simulink model "ideal_buck_boost_non_inverter"  (R2018a)
settings: Solver=FixedStepAuto  StartTime=0.0  StopTime=1  FixedStep=Ti  RelTol=1e-3
undefined symbols (not defined in the file): A, B, Co, disturbance_Ro_enable, disturbance_Ro_time, disturbance_Vin_enable, disturbance_Vin_time, Fsw, L, opt_constant_reference, opt_pwm, opt_theorem, opt_update_equilibrium, P, pwm_limit_lower, pwm_limit_upper, pwm_pid_kd, pwm_pid_ki, pwm_pid_kp, pwm_sample_time, Q, R, Rc, reference_pid_ki, reference_pid_kp, Ro, Ro_p, sensor_sample, sys, Ti, ts, Vo, Vs, Vs_p, xe
libraries: powerlib x19, simulink x6, pePwmGenerator x1
settings Model: SimulationMode=accelerator  Creator=TARCIO-FEM  LastModifiedBy=Julio-LEPO
settings OptimizationCC: EfficientMapNaN2IntZero=off
settings HardwareCC: TargetBitPerPointer=64  TargetBitPerSizeT=64  TargetBitPerPtrDiffT=64  TargetLongLongMode=on  TargetIntDivRoundTo=Zero  TargetEndianess=LittleEndian  TargetWordSize=64  TargetHWDeviceType=MATLAB Host  ProdEqTarget=off
settings CodeAppCC: MaxIdLength=128
settings GRTTargetCC: TargetLangStandard=C89/C90 (ANSI)  CombineOutputUpdateFcns=off  GRTInterface=on

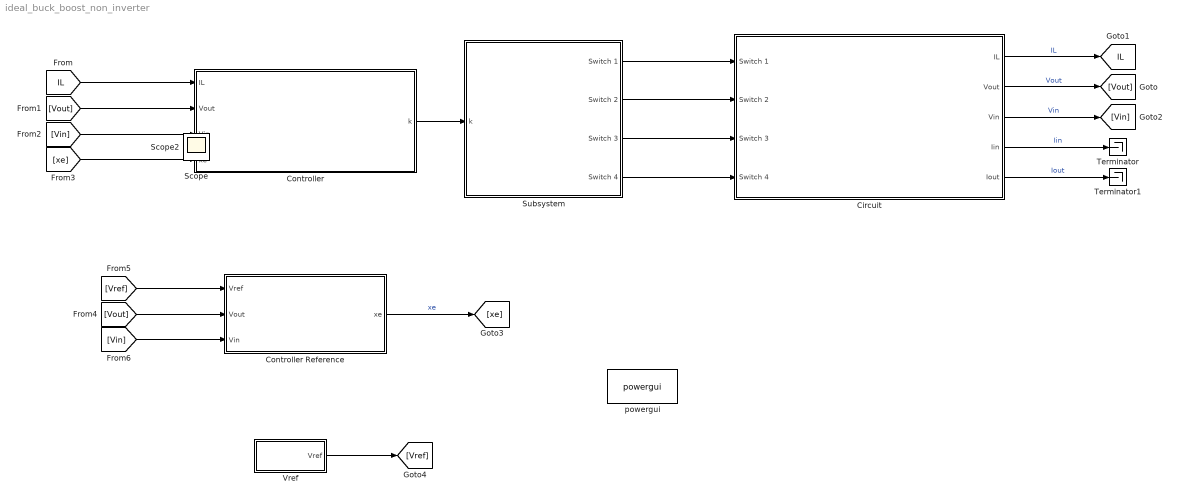
== system ideal_buck_boost_non_inverter ==
  Circuit : Subsystem
  Controller : Subsystem
  Controller Reference : Subsystem
  Subsystem : Subsystem
  Terminator : Terminator
  Terminator1 : Terminator
  Vref : Subsystem
  powergui : powerlib/powergui  Priority=1  SimulationMode=Discrete  SampleTime=Ti  frequency=60  Iterations=50  frequencyindice=0  Pbase=100e6  ErrMax=1e-4  UnitsV=kV  UnitsW=MW  buscounter=0  FunctionMessages=off  echomessages=off  EnableUseOfTLC=off  CurrentSourceSwitches=off  DisableSnubberDevices=off  DisableRonSwitches=off  DisableVfSwitches=off  DisplayEquations=off  SolverType=Tustin/Backward Euler (TBE)  Interpol=off  ExternalGateDelay=off  methode=off  Ts=100  x0status=blocks  SPID=off  SwTol=0  HookPort=off  RestoreLinks=warning  ResistiveCurrentMeasurement=off  Frange=[0:2:500]  Ylog=off  Xlog=on  ShowGrid=off  save=off  variable=ZData  structure=0  ZoomFFT=off  StartTime=0.0  cycles=1  DisplayStyle=1  fundamental=60  FreqAxis=off  MaxFrequency=1000  frequencyindicesteady=1  RmsSteady=1  display=off
  Scope : Scope
  Scope2 : Scope
  tag scope: IL=global
  wires:
  Circuit/1(IL) -> [IL]  "IL"
  Circuit/2(Vout) -> [Vout]  "Vout"
  Circuit/3(Vin) -> [Vin]  "Vin"
  [IL] -> Controller/1(IL)
  [xe] -> Controller/4(xe)
  [Vout] -> Controller Reference/2(Vout)
  [Vin] -> Controller/3(Vin)
  [Vout] -> Controller/2(Vout)
  Controller Reference/1(xe) -> [xe]  "xe"
  [Vin] -> Controller Reference/3(Vin)
  [Vref] -> Controller Reference/1(Vref)
  Vref/1(Vref) -> [Vref]
  Circuit/4(Iin) -> Terminator/1  "Iin"
  Circuit/5(Iout) -> Terminator1/1  "Iout"
  Controller/1(k) -> Subsystem/1(k)
  Subsystem/1(Switch 1) -> Circuit/1(Switch 1)
  Subsystem/2(Switch 2) -> Circuit/2(Switch 2)
  Subsystem/3(Switch 3) -> Circuit/3(Switch 3)
  Subsystem/4(Switch 4) -> Circuit/4(Switch 4)

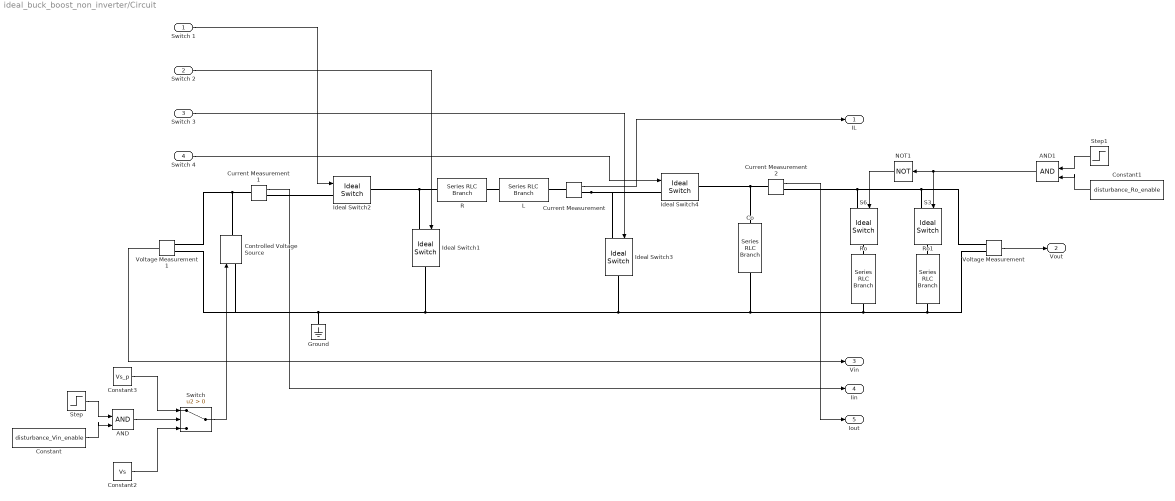
== system ideal_buck_boost_non_inverter/Circuit ==
  Switch 1 : Inport
  Switch 2 : Inport  Port=2
  Switch 3 : Inport  Port=3
  Switch 4 : Inport  Port=4
  AND : Logic  IconShape=distinctive  AllPortsSameDT=off  OutDataTypeStr=boolean
  AND1 : Logic  IconShape=distinctive  AllPortsSameDT=off  OutDataTypeStr=boolean
  Co : powerlib/Elements/Series RLC Branch  LConnTagsString=__new0  RConnTagsString=__new0  BranchType=C  Resistance=Rc  Inductance=L  SetiL0=off  InitialCurrent=0  Capacitance=Co  Setx0=off  InitialVoltage=0  Measurements=None
  Constant : Constant  Value=disturbance_Vin_enable
  Constant1 : Constant  Value=disturbance_Ro_enable
  Constant2 : Constant  Value=Vs
  Constant3 : Constant  Value=Vs_p
  Controlled Voltage Source : powerlib/Electrical Sources/Controlled Voltage Source  Initialize=on  Source_Type=DC  Amplitude=0  Phase=0  Frequency=0  Measurements=None
  Current Measurement : powerlib/Measurements/Current Measurement  PhasorSimulation=off  OutputType=Complex  PSBequivalent=0
  Current Measurement1 : powerlib/Measurements/Current Measurement  PhasorSimulation=off  OutputType=Complex  PSBequivalent=0
  Current Measurement2 : powerlib/Measurements/Current Measurement  PhasorSimulation=off  OutputType=Complex  PSBequivalent=0
  Ground : powerlib/Elements/Ground  LConnTagsString=a
  Ideal Switch{1..4} (4 alike) : powerlib/Power Electronics/Ideal Switch  Ron=0.001  Lon=0  IC=0  Rs=1e5  Cs=inf  Measurements=off
  L : powerlib/Elements/Series RLC Branch  LConnTagsString=__new0  RConnTagsString=__new0  BranchType=L  Resistance=1  Inductance=L  SetiL0=off  InitialCurrent=0  Capacitance=1e-6  Setx0=off  InitialVoltage=0  Measurements=None
  NOT1 : Logic  Operator=NOT  IconShape=distinctive  AllPortsSameDT=off  OutDataTypeStr=boolean
  R : powerlib/Elements/Series RLC Branch  LConnTagsString=__new0  RConnTagsString=__new0  BranchType=R  Resistance=R  Inductance=1e-3  SetiL0=off  InitialCurrent=0  Capacitance=1e-6  Setx0=off  InitialVoltage=0  Measurements=None
  Ro : powerlib/Elements/Series RLC Branch  LConnTagsString=__new0  RConnTagsString=__new0  BranchType=R  Resistance=Ro  Inductance=1e-3  SetiL0=off  InitialCurrent=0  Capacitance=1e-6  Setx0=off  InitialVoltage=0  Measurements=None
  Ro1 : powerlib/Elements/Series RLC Branch  LConnTagsString=__new0  RConnTagsString=__new0  BranchType=R  Resistance=Ro_p  Inductance=1e-3  SetiL0=off  InitialCurrent=0  Capacitance=1e-6  Setx0=off  InitialVoltage=0  Measurements=None
  S3 : powerlib/Power Electronics/Ideal Switch  Ron=0.001  Lon=0  IC=0  Rs=1e5  Cs=inf  Measurements=off
  S6 : powerlib/Power Electronics/Ideal Switch  Ron=0.001  Lon=0  IC=0  Rs=1e5  Cs=inf  Measurements=off
  Step : Step  Time=disturbance_Vin_time  SampleTime=0
  Step1 : Step  Time=disturbance_Ro_time  SampleTime=0
  Switch : Switch  Criteria=u2 > Threshold
  Voltage Measurement : powerlib/Measurements/Voltage Measurement  PhasorSimulation=off  OutputType=Complex  PSBequivalent=0
  Voltage Measurement1 : powerlib/Measurements/Voltage Measurement  PhasorSimulation=off  OutputType=Complex  PSBequivalent=0
  IL : Outport
  Vout : Outport  Port=2
  Vin : Outport  Port=3
  Iin : Outport  Port=4
  Iout : Outport  Port=5
  wires:
  Switch 1/1 -> Ideal Switch2/1
  Voltage Measurement1/1 -> Vin/1
  Voltage Measurement/1 -> Vout/1
  Switch 2/1 -> Ideal Switch1/1
  Constant1/1 -> AND1/2
  AND1/1 -> S3/1, NOT1/1
  NOT1/1 -> S6/1
  Step1/1 -> AND1/1
  AND/1 -> Switch/2
  Constant/1 -> AND/2
  Step/1 -> AND/1
  Constant2/1 -> Switch/3
  Constant3/1 -> Switch/1
  Current Measurement1/1 -> Iin/1
  Current Measurement/1 -> IL/1
  Switch/1 -> Controlled Voltage Source/1
  Current Measurement2/1 -> Iout/1
  Switch 4/1 -> Ideal Switch4/1
  Switch 3/1 -> Ideal Switch3/1
  connections:
  L/LConn1 -- R/RConn1
  Ideal Switch1/LConn1 -- Ideal Switch2/RConn1 -- R/LConn1
  Current Measurement/LConn1 -- L/RConn1
  Current Measurement2/LConn1 -- Ideal Switch4/RConn1 -- Co/LConn1
  Voltage Measurement/LConn2 -- Ro1/RConn1 -- Ro/RConn1 -- Ideal Switch3/RConn1 -- Ideal Switch1/RConn1 -- Voltage Measurement1/LConn2 -- Controlled Voltage Source/LConn1 -- Ground/LConn1 -- Co/RConn1
  S3/RConn1 -- Ro1/LConn1
  S6/RConn1 -- Ro/LConn1
  Current Measurement1/LConn1 -- Controlled Voltage Source/RConn1 -- Voltage Measurement1/LConn1
  Ideal Switch2/LConn1 -- Current Measurement1/RConn1
  S6/LConn1 -- Current Measurement2/RConn1 -- S3/LConn1 -- Voltage Measurement/LConn1
  Current Measurement/RConn1 -- Ideal Switch4/LConn1 -- Ideal Switch3/LConn1

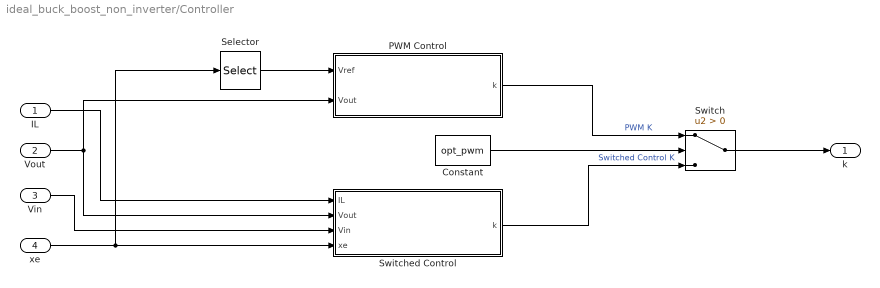
== system ideal_buck_boost_non_inverter/Controller ==
  IL : Inport
  Vout : Inport  Port=2
  Vin : Inport  Port=3
  xe : Inport  Port=4
  Constant : Constant  Value=opt_pwm
  PWM Control : Subsystem
  Selector : Selector  InputPortWidth=2  IndexOptions=Index vector (dialog)  Indices=[2]  OutputSizes=1
  Switch : Switch  Criteria=u2 > Threshold
  Switched Control : Subsystem
  k : Outport
  wires:
  IL/1 -> Switched Control/1(IL)
  Vout/1 -> PWM Control/2(Vout), Switched Control/2(Vout)
  Vin/1 -> Switched Control/3(Vin)
  Switch/1 -> k/1
  PWM Control/1(k) -> Switch/1  "PWM K"
  Switched Control/1(k) -> Switch/3  "Switched Control K"
  Constant/1 -> Switch/2
  xe/1 -> Selector/1, Switched Control/4(xe)
  Selector/1 -> PWM Control/1(Vref)

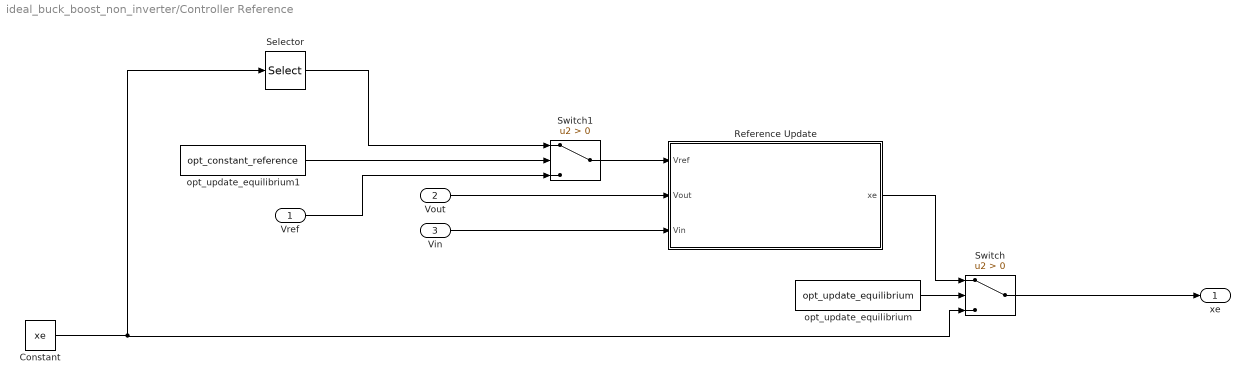
== system ideal_buck_boost_non_inverter/Controller Reference ==
  Vref : Inport
  Vout : Inport  Port=2
  Vin : Inport  Port=3
  Constant : Constant  Value=xe
  Reference Update : Subsystem
  Selector : Selector  InputPortWidth=2  IndexOptions=Index vector (dialog)  Indices=[2]  OutputSizes=1
  Switch : Switch  Criteria=u2 > Threshold
  Switch1 : Switch  Criteria=u2 > Threshold
  opt_update_equilibrium : Constant  Value=opt_update_equilibrium
  opt_update_equilibrium1 : Constant  Value=opt_constant_reference
  xe : Outport
  wires:
  Reference Update/1(xe) -> Switch/1
  opt_update_equilibrium/1 -> Switch/2
  Vout/1 -> Reference Update/2(Vout)
  Constant/1 -> Switch/3, Selector/1
  Vin/1 -> Reference Update/3(Vin)
  Switch/1 -> xe/1
  Switch1/1 -> Reference Update/1(Vref)
  Selector/1 -> Switch1/1
  Vref/1 -> Switch1/3
  opt_update_equilibrium1/1 -> Switch1/2

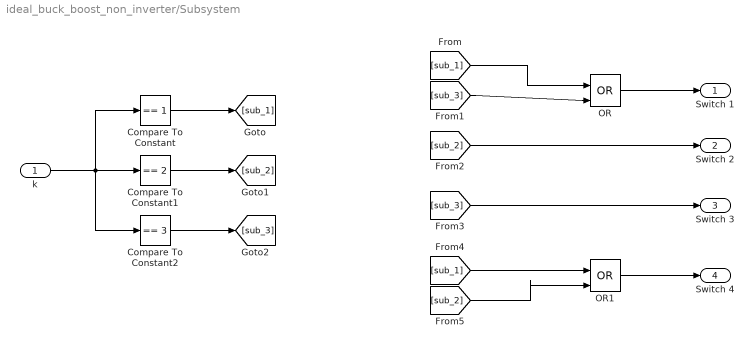
== system ideal_buck_boost_non_inverter/Subsystem ==
  k : Inport
  Compare To Constant : simulink/Logic and Bit Operations/Compare To Constant  relop===  const=1  OutDataTypeStr=boolean
  Compare To Constant1 : simulink/Logic and Bit Operations/Compare To Constant  relop===  const=2  OutDataTypeStr=boolean
  Compare To Constant2 : simulink/Logic and Bit Operations/Compare To Constant  relop===  const=3  OutDataTypeStr=boolean
  OR : Logic  Operator=OR  IconShape=distinctive  AllPortsSameDT=off  OutDataTypeStr=boolean
  OR1 : Logic  Operator=OR  IconShape=distinctive  AllPortsSameDT=off  OutDataTypeStr=boolean
  Switch 1 : Outport
  Switch 2 : Outport  Port=2
  Switch 3 : Outport  Port=3
  Switch 4 : Outport  Port=4
  wires:
  OR/1 -> Switch 1/1
  k/1 -> Compare To Constant2/1, Compare To Constant1/1, Compare To Constant/1
  Compare To Constant/1 -> [sub_1]
  Compare To Constant2/1 -> [sub_3]
  Compare To Constant1/1 -> [sub_2]
  [sub_1] -> OR/1
  [sub_3] -> OR/2
  [sub_2] -> Switch 2/1
  [sub_3] -> Switch 3/1
  [sub_1] -> OR1/1
  [sub_2] -> OR1/2
  OR1/1 -> Switch 4/1

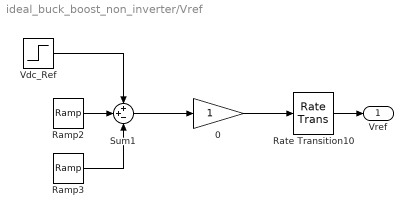
== system ideal_buck_boost_non_inverter/Vref ==
  0 : Gain
  Ramp2 : simulink/Sources/Ramp  slope=Vo/ts  start=0  InitialOutput=0
  Ramp3 : simulink/Sources/Ramp  slope=Vo/ts  start=ts  InitialOutput=0
  Rate Transition10 : RateTransition  OutPortSampleTimeOpt=Inherit  OutPortSampleTime=Ts
  Sum1 : Sum  Inputs=++-
  Vdc_Ref : Step  Time=0.3  After=10  SampleTime=0
  Vref : Outport
  wires:
  Ramp2/1 -> Sum1/2
  Ramp3/1 -> Sum1/3
  0/1 -> Rate Transition10/1
  Sum1/1 -> 0/1
  Vdc_Ref/1 -> Sum1/1
  Rate Transition10/1 -> Vref/1

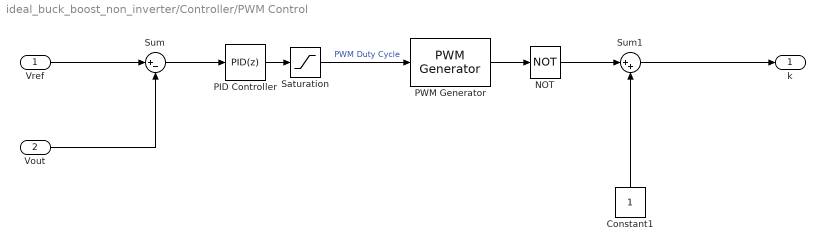
== system ideal_buck_boost_non_inverter/Controller/PWM Control ==
  Vref : Inport
  Vout : Inport  Port=2
  Constant1 : Constant
  NOT : Logic  Operator=NOT  IconShape=distinctive  AllPortsSameDT=off  OutDataTypeStr=boolean
  PID Controller : simulink/Continuous/PID Controller  Controller=PID  TimeDomain=Discrete-time  SampleTime=sensor_sample  IntegratorMethod=Forward Euler  FilterMethod=Forward Euler  Form=Parallel  UseFilter=on  ControllerParametersSource=internal  P=pwm_pid_kp  I=pwm_pid_ki  D=pwm_pid_kd  N=100  InitialConditionSource=internal  InitialConditionForIntegrator=0  InitialConditionForFilter=0  ExternalReset=none  LimitOutput=off  UpperSaturationLimit=inf  LowerSaturationLimit=-inf  LinearizeAsGain=on  AntiWindupMode=none  Kb=1  TrackingMode=off  Kt=1  PParamMin=[]  PParamMax=[]  IParamMin=[]  IParamMax=[]  DParamMin=[]  DParamMax=[]  NParamMin=[]  NParamMax=[]  KbParamMin=[]  KbParamMax=[]  KtParamMin=[]  KtParamMax=[]  POutMin=[]  POutMax=[]  IOutMin=[]  IOutMax=[]  DOutMin=[]  DOutMax=[]  NOutMin=[]  NOutMax=[]  KbOutMin=[]  KbOutMax=[]  KtOutMin=[]  KtOutMax=[]  IntegratorOutMin=[]  IntegratorOutMax=[]  FilterOutMin=[]  FilterOutMax=[]  SumOutMin=[]  SumOutMax=[]  SumI1OutMin=[]  SumI1OutMax=[]  SumI2OutMin=[]  SumI2OutMax=[]  SumI3OutMin=[]  SumI3OutMax=[]  SumDOutMin=[]  SumDOutMax=[]  SaturationOutMin=[]  SaturationOutMax=[]  IntegratorContinuousStateAttributes=''  IntegratorStateMustResolveToSignalObject=off  IntegratorRTWStateStorageClass=Auto  FilterContinuousStateAttributes=''  FilterStateMustResolveToSignalObject=off  FilterRTWStateStorageClass=Auto  DifferentiatorICPrevScaledInput=0  DifferentiatorOutMin=[]  DifferentiatorOutMax=[]  FilterDiffOutCoefMin=[]  FilterDiffOutCoefMax=[]  SumDenOutMin=[]  SumDenOutMax=[]  SumNumOutMin=[]  SumNumOutMax=[]  ReciprocalOutMin=[]  ReciprocalOutMax=[]  DivideOutMin=[]  DivideOutMax=[]  TunerSelectOption=Transfer Function Based (PID Tuner App)
  PWM Generator : pePwmGenerator/PWM Generator  CarrCount=Up  Tper=pwm_period  Ts=pwm_sample_time
  Saturation : Saturate  UpperLimit=pwm_limit_upper  LowerLimit=pwm_limit_lower
  Sum : Sum  Inputs=|+-
  Sum1 : Sum  Inputs=|++
  k : Outport
  wires:
  PWM Generator/1 -> NOT/1
  PID Controller/1 -> Saturation/1
  Saturation/1 -> PWM Generator/1  "PWM Duty Cycle"
  Sum/1 -> PID Controller/1
  Vref/1 -> Sum/1
  Sum1/1 -> k/1
  Vout/1 -> Sum/2
  NOT/1 -> Sum1/1
  Constant1/1 -> Sum1/2

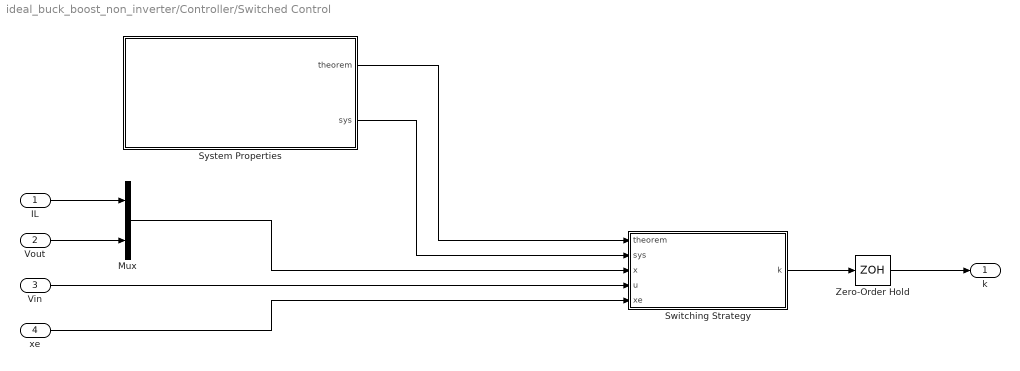
== system ideal_buck_boost_non_inverter/Controller/Switched Control ==
  IL : Inport
  Vout : Inport  Port=2
  Vin : Inport  Port=3
  xe : Inport  Port=4
  Mux : Mux  Inputs=2
  Switching Strategy : MATLAB Function  TreatAsAtomicUnit=on
  System Properties : Subsystem
  Zero-Order Hold : ZeroOrderHold  SampleTime=1/Fsw
  k : Outport
  wires:
  Vin/1 -> Switching Strategy/4(u)
  Switching Strategy/1(k) -> Zero-Order Hold/1
  System Properties/1(theorem) -> Switching Strategy/1(theorem)
  System Properties/2(sys) -> Switching Strategy/2(sys)
  Mux/1 -> Switching Strategy/3(x)
  IL/1 -> Mux/1
  Vout/1 -> Mux/2
  xe/1 -> Switching Strategy/5(xe)
  Zero-Order Hold/1 -> k/1

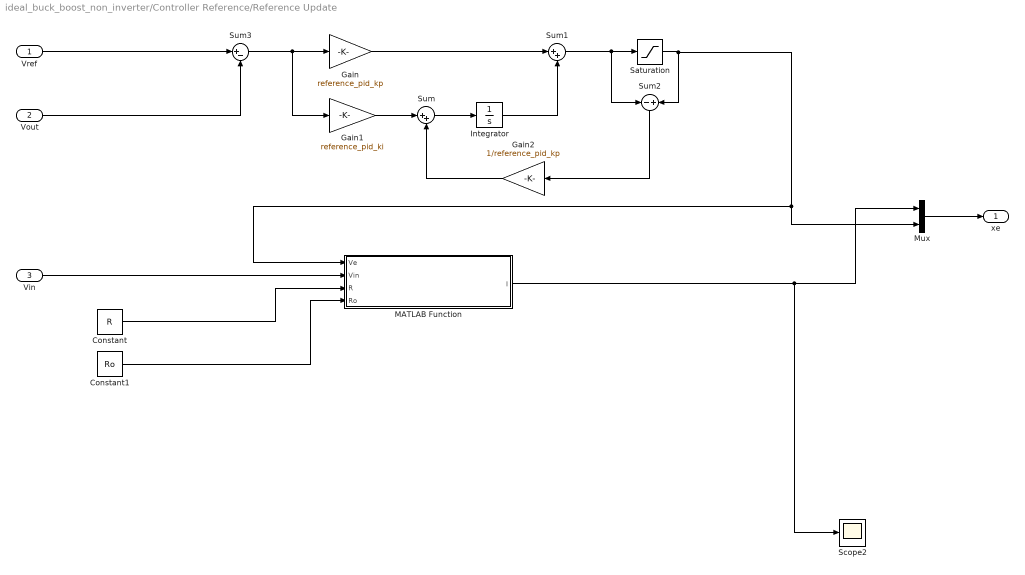
== system ideal_buck_boost_non_inverter/Controller Reference/Reference Update ==
  Vref : Inport
  Vout : Inport  Port=2
  Vin : Inport  Port=3
  Constant : Constant  Value=R
  Constant1 : Constant  Value=Ro
  Gain : Gain  Gain=reference_pid_kp
  Gain1 : Gain  Gain=reference_pid_ki
  Gain2 : Gain  Gain=1/reference_pid_kp
  Integrator : Integrator
  MATLAB Function : MATLAB Function  TreatAsAtomicUnit=on
  Mux : Mux  Inputs=2
  Saturation : Saturate  UpperLimit=400  LowerLimit=0
  Scope2 : Scope
  Sum : Sum  Inputs=|++
  Sum1 : Sum  Inputs=|++
  Sum2 : Sum  Inputs=-|+
  Sum3 : Sum  Inputs=|+-
  xe : Outport
  wires:
  Gain1/1 -> Sum/1
  Gain2/1 -> Sum/2
  Sum/1 -> Integrator/1
  Gain/1 -> Sum1/1
  Integrator/1 -> Sum1/2
  Sum1/1 -> Sum2/1, Saturation/1
  Sum2/1 -> Gain2/1
  Sum3/1 -> Gain1/1, Gain/1
  Vref/1 -> Sum3/1
  Vout/1 -> Sum3/2
  Mux/1 -> xe/1
  Saturation/1 -> Mux/2, MATLAB Function/1(Ve), Sum2/2
  Vin/1 -> MATLAB Function/2(Vin)
  MATLAB Function/1(I) -> Mux/1, Scope2/1
  Constant/1 -> MATLAB Function/3(R)
  Constant1/1 -> MATLAB Function/4(Ro)

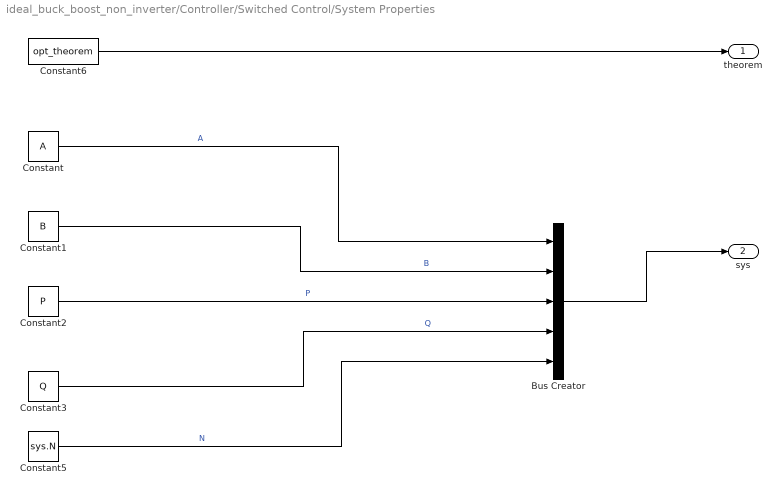
== system ideal_buck_boost_non_inverter/Controller/Switched Control/System Properties ==
  Bus Creator : BusCreator  Inputs=5  OutDataTypeStr=Bus: SystemDataBus
  Constant : Constant  Value=A  VectorParams1D=off
  Constant1 : Constant  Value=B  VectorParams1D=off
  Constant2 : Constant  Value=P  VectorParams1D=off
  Constant3 : Constant  Value=Q  VectorParams1D=off
  Constant5 : Constant  Value=sys.N
  Constant6 : Constant  Value=opt_theorem
  theorem : Outport
  sys : Outport  Port=2
  wires:
  Bus Creator/1 -> sys/1
  Constant2/1 -> Bus Creator/3  "P"
  Constant1/1 -> Bus Creator/2  "B"
  Constant/1 -> Bus Creator/1  "A"
  Constant3/1 -> Bus Creator/4  "Q"
  Constant5/1 -> Bus Creator/5  "N"
  Constant6/1 -> theorem/1

== matlab function ideal_buck_boost_non_inverter/Controller Reference/Reference Update/MATLAB Function ==
  data: Ve input; I output; Vin input; R input; Ro input
function I = EquilibriumCurrent(Ve, Vin, R, Ro)
    I = Ve/Ro;
end

== matlab function ideal_buck_boost_non_inverter/Controller/Switched Control/Switching Strategy ==
  data: theorem input; sys input; x input; u input; k output; xe input
function k = switching_strategy(theorem, sys, x, u, xe)
    qsi = x - xe;
    sig = zeros(sys.N,1);
    
    for i=1:sys.N
        switch(theorem)
            case 1
                sig(i) = qsi'*(sys.Q(:,:,i)*qsi + 2*sys.P*(sys.A(:,:,i)*x + sys.B(:,:,i)*u));
            case 2
                sig(i) = qsi'*sys.P*(sys.A(:,:,i)*xe + sys.B(:,:,i)*u);
        end
    end
    [~, k] = min(sig);
end
